simulink model "chap2_2sim"  (R2016a)
settings: Solver=ode45  StartTime=0.0  StopTime=2000  RelTol=1e-3
settings Model: Creator=zhanghankui  LastModifiedBy=zhanghankui
settings DataIOCC: SaveOutput=off  SignalLogging=off  DSMLogging=off  SaveTime=off

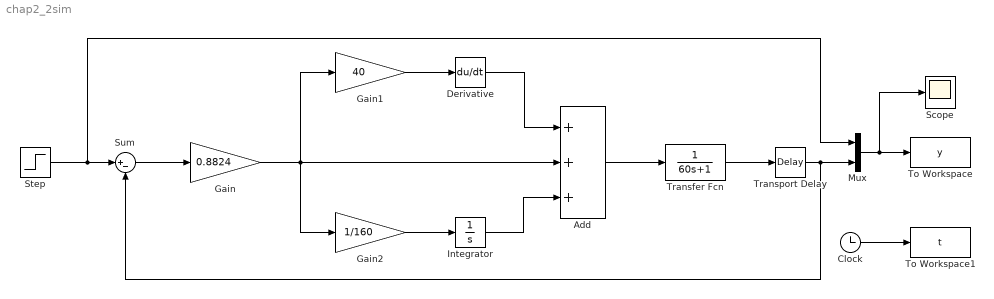
== system chap2_2sim ==
  Add : Sum  Inputs=3
  Clock : Clock
  Derivative : Derivative
  Gain : Gain  Gain=0.8824
  Gain1 : Gain  Gain=40
  Gain2 : Gain  Gain=1/160
  Integrator : Integrator
  Mux : Mux  Inputs=2
  Scope : Scope
  Step : Step  Time=0  SampleTime=0
  Sum : Sum  Inputs=|+-
  To Workspace : ToWorkspace  VariableName=y  SampleTime=-1
      settings: Save2DSignal=2-D array (concatenate along first dimension)
  To Workspace1 : ToWorkspace  VariableName=t  SampleTime=-1
      settings: Save2DSignal=2-D array (concatenate along first dimension)
  Transfer Fcn : TransferFcn  Denominator=[60 1]
  Transport Delay : TransportDelay  DelayTime=80
  wires:
  Step/1 -> Mux/1, Sum/1
  Sum/1 -> Gain/1
  Gain2/1 -> Integrator/1
  Gain1/1 -> Derivative/1
  Gain/1 -> Gain2/1, Gain1/1, Add/2
  Derivative/1 -> Add/1
  Integrator/1 -> Add/3
  Add/1 -> Transfer Fcn/1
  Transfer Fcn/1 -> Transport Delay/1
  Transport Delay/1 -> Sum/2, Mux/2
  Mux/1 -> Scope/1, To Workspace/1
  Clock/1 -> To Workspace1/1
